simulink model "UnitDelaySubSystem3Layers"  (Simulink 7.6)
settings: Solver=ode45  StartTime=0.0  StopTime=10.0  RelTol=1e-3
settings Model: Creator=DominikC  LastModifiedBy=DominikC
settings DebuggingCC: FcnCallInpInsideContextMsg=Enable All

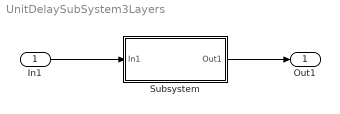
== system UnitDelaySubSystem3Layers ==
  In1 : Inport
  Subsystem : Subsystem
  Out1 : Outport
  wires:
  In1/1 -> Subsystem/1(In1)
  Subsystem/1(Out1) -> Out1/1

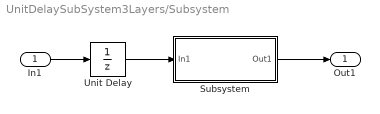
== system UnitDelaySubSystem3Layers/Subsystem ==
  In1 : Inport
  Subsystem : Subsystem
  Unit Delay : UnitDelay  SampleTime=-1
  Out1 : Outport
  wires:
  In1/1 -> Unit Delay/1
  Unit Delay/1 -> Subsystem/1(In1)
  Subsystem/1(Out1) -> Out1/1

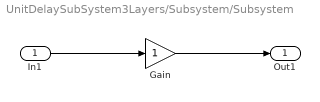
== system UnitDelaySubSystem3Layers/Subsystem/Subsystem ==
  In1 : Inport
  Gain : Gain
  Out1 : Outport
  wires:
  In1/1 -> Gain/1
  Gain/1 -> Out1/1
